simulink model "neuromuscular_reflex_sim"  (R2021b)
settings: Solver=VariableStepAuto  StartTime=0.0  StopTime=10.0  RelTol=1e-3
values from neighbouring files (symbols this model uses):
  b_m = 2    [neuromuscular_reflex.m]
  b_s = 1    [neuromuscular_reflex.m]
  beta = 100    [neuromuscular_reflex.m]
  k_m = 50    [neuromuscular_reflex.m]
  k_s1 = 240    [neuromuscular_reflex.m]
  k_s2 = 60    [neuromuscular_reflex.m]
  m = 0.1    [neuromuscular_reflex.m]
undefined symbols (not defined in the file or in its folder): sigbuilder_block
settings Model: Creator=eraym  LastModifiedBy=eraym

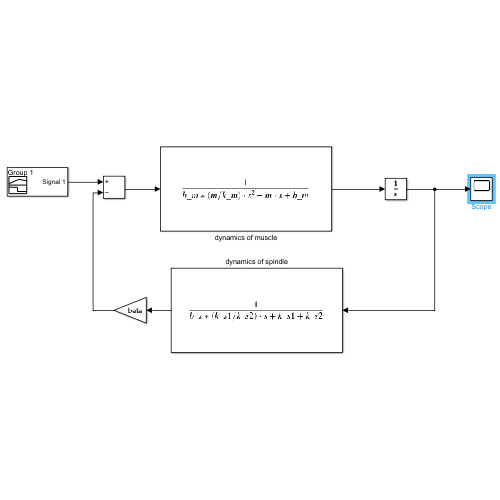
[thumbnail: Simulink's stored preview of the top-level diagram]
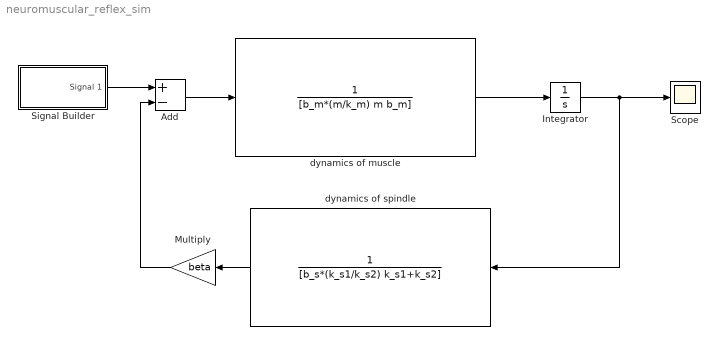
== system neuromuscular_reflex_sim ==
  Add : Sum  Inputs=+-
  Integrator : Integrator
  Multiply : Gain  Gain=beta
  Scope : Scope
  Signal Builder : Subsystem  Tag=STV Subsys  LoadFcn=sigbuilder_block('load');  StartFcn=sigbuilder_block('start');  StopFcn=sigbuilder_block('stop');  ClipboardFcn=sigbuilder_block('clipboard');  mask(Sigbuilder block){tuvar=[0:10]}
      mask help: Simulink:masks:SigbuilderBlock_MD
      mask init:
      | if ~strcmp(get_param(bdroot(gcbh),'SimulationStatus'),'stopped') tuvar = sigbuilder_block('maskInit'); end
      settings: CopyFcn=sigbuilder_block('copy');  DeleteFcn=sigbuilder_block('delete');  ModelCloseFcn=sigbuilder_block('modelClose');  PreSaveFcn=sigbuilder_block('preSave');  PauseFcn=sigbuilder_block('pause');  ContinueFcn=sigbuilder_block('continue');  NameChangeFcn=sigbuilder_block('namechange');  OpenFcn=sigbuilder_block('open',[437.6 199.2 550.4 400 ]);  CloseFcn=sigbuilder_block('close');
      mask Display: plot(0, 0, 100, 100,[2, 2, 32, 32, 2], [68, 8, 8, 68, 68],[32, 2], [38, 38], [32, 19, 2],[53, 60, 44], [32, 17, 17, 2],[16, 16, 31, 31]);txt = getActiveGroup(gcbh);text(2, 100, txt,'verticalAlignment', 'top');
  dynamics of muscle : TransferFcn  Denominator=[b_m*(m/k_m) m b_m]
  dynamics of spindle : TransferFcn  Denominator=[b_s*(k_s1/k_s2) k_s1+k_s2]
  wires:
  Signal Builder/1(Signal 1) -> Add/1
  Multiply/1 -> Add/2
  Add/1 -> dynamics of muscle/1
  dynamics of muscle/1 -> Integrator/1
  dynamics of spindle/1 -> Multiply/1
  Integrator/1 -> Scope/1, dynamics of spindle/1

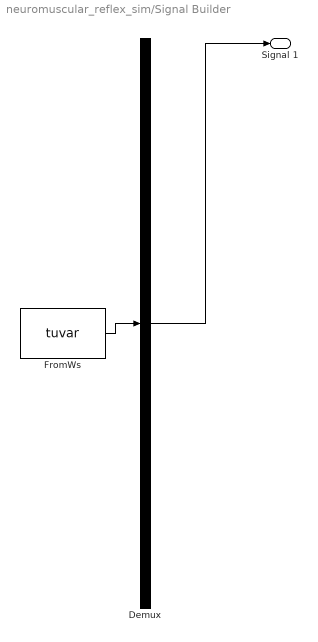
== system neuromuscular_reflex_sim/Signal Builder ==
  Demux : Demux  Tag=STV Demux  Outputs=1
      settings: DisplayOption=none
  FromWs : FromWorkspace  Tag=STV FromWs  VariableName=tuvar
      SigBuilderData=|
      | common.afterFinalStr = 'Extrapolate'
      | common.sampleTime = 0
      | dataSet.timeRange = [0 10]
      | dataSet.name = 'Group 1'
      | sbobj.Groups.Name = 'Group 1'
      | sbobj.Groups.Signals.Name = 'Signal 1'
      | sbobj.Groups.Signals.XData = [0 1.98 1.98 3 3 10]
      | sbobj.Groups.Signals.YData = [0 0 1 1 0 0]
  Signal 1 : Outport  Tag=STV Outport
  wires:
  Demux/1 -> Signal 1/1
  FromWs/1 -> Demux/1
